simulink model "vrtut3"  (R2014a)
settings: Solver=ode45  StartTime=0.0  StopTime=Inf  RelTol=1e-3
libraries: vrlib x3
Description:
  | Simulink(R) 3D Animation(TM) - Tutorial #3
  | 
  | Tutorial model to be used for 3D World Editor authoring example in the documentation.
  | After creating the virtual world according to the instructions in the documentation, include the VR block
  | in the model and connect B1, B2 coordinates and S scaling to corresponding nodes in
  | the virtual world.
settings Model: CovMetricSettings=d  ExtModeTrigMode=oneshot  ExtModeArmWhenConnect=off  Creator=Danek  LastModifiedBy=gxnuhuang
settings DataIOCC: SignalLoggingSaveFormat=ModelDataLogs  SaveOutput=off  SaveTime=off  SignalLoggingName=logsOut
settings OptimizationCC: BooleanDataType=off  ExpressionDepthLimit=2147483647  InitFltsAndDblsToZero=on
settings DebuggingCC: UnderspecifiedInitializationDetection=Classic  CheckExecutionContextPreStartOutputMsg=on  CheckExecutionContextRuntimeOutputMsg=on  SignalResolutionControl=TryResolveAllWithWarning  SolverPrmCheckMsg=none  MultiTaskDSMMsg=warning  MultiTaskCondExecSysMsg=none  FcnCallInpInsideContextMsg=UseLocalSettings  StateNameClashWarn=warning  StrictBusMsg=None
settings HardwareCC: TargetUnknown=on
settings ModelReferenceCC: UpdateModelReferenceTargets=IfOutOfDate
settings RTWCC: IncludeERTFirstTime=on
settings GRTTargetCC: TargetFcnLib=ansi_tfl_tmw.mat  CombineOutputUpdateFcns=off  GRTInterface=on

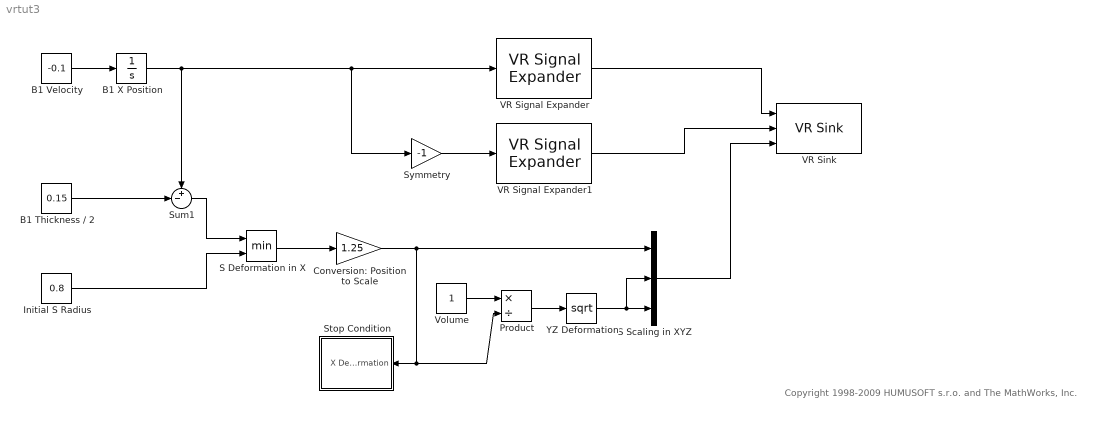
== system vrtut3 ==
  note: Copyright 1998-2009 HUMUSOFT s.r.o. and The MathWorks, Inc.
  B1 Thickness / 2 : Constant  Value=0.15
  B1 Velocity : Constant  Value=-0.1
  B1 X Position : Integrator  InitialCondition=3  UpperSaturationLimit=Inf  LowerSaturationLimit=-Inf
  Conversion: Position to Scale : Gain  Gain=1.25  SaturateOnIntegerOverflow=on  OutDataTypeStr=Inherit: Same as input  ParamDataTypeStr=Inherit: Same as input
  Initial S Radius : Constant  Value=0.8
  Product : Product  Inputs=*/  SaturateOnIntegerOverflow=on  RndMeth=Zero  InputSameDT=on  OutDataTypeStr=Inherit: Same as first input
  "S Deformation in X " : MinMax  Inputs=2  SaturateOnIntegerOverflow=on  InputSameDT=on
  S Scaling in XYZ : Mux  Inputs=3
  Stop Condition : Subsystem
  Sum1 : Sum  Inputs=+-|  SaturateOnIntegerOverflow=on  InputSameDT=on  OutDataTypeStr=Inherit: Same as first input
  Symmetry : Gain  Gain=-1  SaturateOnIntegerOverflow=on  OutDataTypeStr=Inherit: Same as input  ParamDataTypeStr=Inherit: Same as input
  VR Signal Expander : vrlib/VR Signal Expander  outwidth=3  outidx=1
  VR Signal Expander1 : vrlib/VR Signal Expander  outwidth=3  outidx=1
  VR Sink : vrlib/VR Sink  InstantiateOnLoad=on  SampleTime=0.1  ViewEnable=on  RemoteChange=off  RemoteView=off  FieldsWritten=B1.translation.3.1.1.double#B2.translation.3.1.1.double#S.scale.3.1.1.double  WorldFileName=vrtut3.wrl  WorldDescription=vrtut3  AutoView=on  VideoDimensions=[]  AllowVariableSize=off
  Volume : Constant
  YZ Deformation : Math  Operator=sqrt  SaturateOnIntegerOverflow=on
  wires:
  Symmetry/1 -> VR Signal Expander1/1
  B1 X Position/1 -> Symmetry/1, VR Signal Expander/1, Sum1/1
  "S Deformation in X "/1 -> Conversion: Position to Scale/1
  B1 Velocity/1 -> B1 X Position/1
  B1 Thickness / 2/1 -> Sum1/2
  Initial S Radius/1 -> "S Deformation in X "/2
  Sum1/1 -> "S Deformation in X "/1
  Conversion: Position to Scale/1 -> Product/2, Stop Condition/1(X Deformation), S Scaling in XYZ/1
  Volume/1 -> Product/1
  Product/1 -> YZ Deformation/1
  YZ Deformation/1 -> S Scaling in XYZ/2, S Scaling in XYZ/3
  S Scaling in XYZ/1 -> VR Sink/3
  VR Signal Expander/1 -> VR Sink/1
  VR Signal Expander1/1 -> VR Sink/2

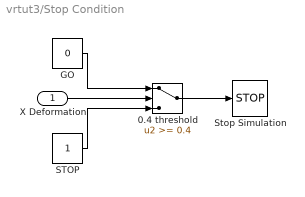
== system vrtut3/Stop Condition ==
  X Deformation : Inport
  0.4 threshold : Switch  Threshold=0.4  SaturateOnIntegerOverflow=on  InputSameDT=on
  GO : Constant  Value=0
  STOP : Constant
  Stop Simulation : Stop
  wires:
  X Deformation/1 -> 0.4 threshold/2
  GO/1 -> 0.4 threshold/1
  STOP/1 -> 0.4 threshold/3
  0.4 threshold/1 -> Stop Simulation/1
